simulink model "URM_IOKU_trajektorie_4_pokus"  (R2014a)
settings: Solver=ode45  StartTime=0.0  StopTime=3.975  MaxStep=1e-2  RelTol=1e-3
values from neighbouring files (symbols this model uses):
  a1 = 2    [URM_SP.m]
  a2 = 1.5    [URM_SP.m]
  a3 = 0.5    [URM_SP.m]
  D = linspace(d1,d2,n)    [URM_SP.m]
  vmax = 1    [URM_SP.m]
libraries: mblibv1 x12
settings Model: Creator=kajak_000  LastModifiedBy=kajak_000
settings SimMechanicsCC: VisDuringSimulation=on

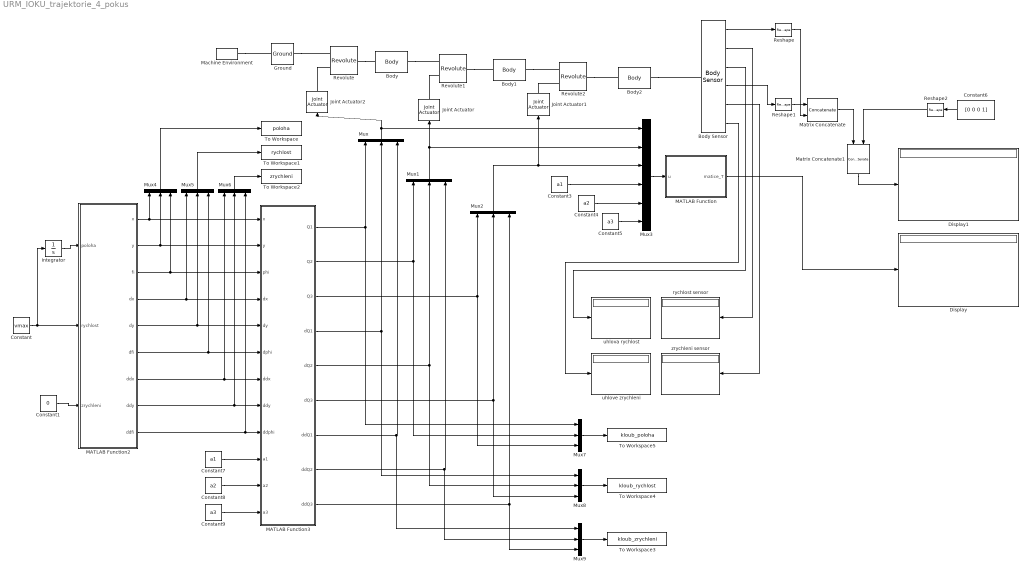
== system URM_IOKU_trajektorie_4_pokus ==
  Body : mblibv1/Bodies/Body  LConnTagsString=CS1  RConnTagsString=CS2  UpdateFromCAD=off  DialogClass=MechanicalBodyBlock  Mass=1  MassUnits=kg  InertiaUnits=kg*m^2  Inertia=eye(3)  Shape=Cylinder  ShapeDims=[1 1]  ShapeUnits=m  ShapeUse=false  Density=1  DensityUnits=kg/m^3  DensityUse=false  GraphicsMode=MACHINE_DEFAULT  BodyColorSelMode=MACHINE_DEFAULT  BodyColor=[1 0 0]  AttachedToCS=CG  CG=Left$CG$rameno1.CG$WORLD$WORLD$m$[0 0 0]$Euler X-Y-Z$deg$WORLD$false$none  WorkingFrames=Left$CS1$rameno1.A$World$World$m$[0 0 0]$Euler X-Y-Z$deg$WORLD$true$none#Right$CS2$rameno1.B$World$World$m$[0 0 0]$Euler X-Y-Z$deg$WORLD$true$none  CGPos=rameno1.CG  CGRot=[0 0 0]  CS0Pos=[]  CS0Rot=[]  CS1Pos=rameno1.A  CS1Rot=[0 0 0]  CS2Pos=rameno1.B  CS2Rot=[0 0 0]  CS3Pos=[]  CS3Rot=[]  CS4Pos=[]  CS4Rot=[]  CS5Pos=[]  CS5Rot=[]  CS6Pos=[]  CS6Rot=[]  CS7Pos=[]  CS7Rot=[]  CS8Pos=[]  CS8Rot=[]  CS9Pos=[]  CS9Rot=[]  CS10Pos=[]  CS10Rot=[]  CS11Pos=[]  CS11Rot=[]  CS12Pos=[]  CS12Rot=[]  CS13Pos=[]  CS13Rot=[]  CS14Pos=[]  CS14Rot=[]  CS15Pos=[]  CS15Rot=[]  CS16Pos=[]  CS16Rot=[]  CS17Pos=[]  CS17Rot=[]  CS18Pos=[]  CS18Rot=[]  CS19Pos=[]  CS19Rot=[]  CS20Pos=[]  CS20Rot=[]
  Body Sensor : mblibv1/Sensors &  Actuators/Body Sensor  UpdateFromCAD=off  PhysicalDomain=Mechanical  PortType=blob  Muxed=off  Pose=on  Angle=on  AngleUnits=deg  ArcVelocity=on  ArcVelocityUnits=rad/s  ArcAcceleration=on  ArcAccelerationUnits=rad/s^2  CoordPosition=on  CoordPositionUnits=m  Velocity=on  VelocityUnits=m/s  Acceleration=on  AccelerationUnits=m/s^2  Quaternion=on  QuaternionDT=off  QuaternionDDT=off  QuaternionUnits=off  OutputVector="[ 3  3  3  9  3  3]"  ActiveIO=on  Width=24  DialogClass=MechanicalSensorBlock  ReferenceFrame=Absolute (World)
  Body1 : mblibv1/Bodies/Body  LConnTagsString=CS1  RConnTagsString=CS2  UpdateFromCAD=off  DialogClass=MechanicalBodyBlock  Mass=1  MassUnits=kg  InertiaUnits=kg*m^2  Inertia=eye(3)  Shape=Cylinder  ShapeDims=[1 1]  ShapeUnits=m  ShapeUse=false  Density=1  DensityUnits=kg/m^3  DensityUse=false  GraphicsMode=MACHINE_DEFAULT  BodyColorSelMode=MACHINE_DEFAULT  BodyColor=[1 0 0]  AttachedToCS=CG  CG=Left$CG$rameno2.CG$WORLD$WORLD$m$[0 0 0]$Euler X-Y-Z$deg$WORLD$false$none  WorkingFrames=Left$CS1$rameno2.A$World$World$m$[0 0 0]$Euler X-Y-Z$deg$WORLD$true$none#Right$CS2$rameno2.B$World$World$m$[0 0 0]$Euler X-Y-Z$deg$WORLD$true$none  CGPos=rameno2.CG  CGRot=[0 0 0]  CS0Pos=[]  CS0Rot=[]  CS1Pos=rameno2.A  CS1Rot=[0 0 0]  CS2Pos=rameno2.B  CS2Rot=[0 0 0]  CS3Pos=[]  CS3Rot=[]  CS4Pos=[]  CS4Rot=[]  CS5Pos=[]  CS5Rot=[]  CS6Pos=[]  CS6Rot=[]  CS7Pos=[]  CS7Rot=[]  CS8Pos=[]  CS8Rot=[]  CS9Pos=[]  CS9Rot=[]  CS10Pos=[]  CS10Rot=[]  CS11Pos=[]  CS11Rot=[]  CS12Pos=[]  CS12Rot=[]  CS13Pos=[]  CS13Rot=[]  CS14Pos=[]  CS14Rot=[]  CS15Pos=[]  CS15Rot=[]  CS16Pos=[]  CS16Rot=[]  CS17Pos=[]  CS17Rot=[]  CS18Pos=[]  CS18Rot=[]  CS19Pos=[]  CS19Rot=[]  CS20Pos=[]  CS20Rot=[]
  Body2 : mblibv1/Bodies/Body  LConnTagsString=CS1  RConnTagsString=CS2  UpdateFromCAD=off  DialogClass=MechanicalBodyBlock  Mass=1  MassUnits=kg  InertiaUnits=kg*m^2  Inertia=eye(3)  Shape=Cylinder  ShapeDims=[1 1]  ShapeUnits=m  ShapeUse=false  Density=1  DensityUnits=kg/m^3  DensityUse=false  GraphicsMode=MACHINE_DEFAULT  BodyColorSelMode=MACHINE_DEFAULT  BodyColor=[1 0 0]  AttachedToCS=CG  CG=Left$CG$rameno3.CG$WORLD$WORLD$m$[0 0 0]$Euler X-Y-Z$deg$WORLD$false$none  WorkingFrames=Left$CS1$rameno3.A$World$World$m$[0 0 0]$Euler X-Y-Z$deg$WORLD$true$none#Right$CS2$rameno3.B$World$World$m$[0 0 0]$Euler X-Y-Z$deg$WORLD$true$none  CGPos=rameno3.CG  CGRot=[0 0 0]  CS0Pos=[]  CS0Rot=[]  CS1Pos=rameno3.A  CS1Rot=[0 0 0]  CS2Pos=rameno3.B  CS2Rot=[0 0 0]  CS3Pos=[]  CS3Rot=[]  CS4Pos=[]  CS4Rot=[]  CS5Pos=[]  CS5Rot=[]  CS6Pos=[]  CS6Rot=[]  CS7Pos=[]  CS7Rot=[]  CS8Pos=[]  CS8Rot=[]  CS9Pos=[]  CS9Rot=[]  CS10Pos=[]  CS10Rot=[]  CS11Pos=[]  CS11Rot=[]  CS12Pos=[]  CS12Rot=[]  CS13Pos=[]  CS13Rot=[]  CS14Pos=[]  CS14Rot=[]  CS15Pos=[]  CS15Rot=[]  CS16Pos=[]  CS16Rot=[]  CS17Pos=[]  CS17Rot=[]  CS18Pos=[]  CS18Rot=[]  CS19Pos=[]  CS19Rot=[]  CS20Pos=[]  CS20Rot=[]
  Constant : Constant  Value=vmax
  Constant1 : Constant  Value=0
  Constant3 : Constant  Value=a1
  Constant4 : Constant  Value=a2
  Constant5 : Constant  Value=a3
  Constant6 : Constant  Value=[0 0 0 1]
  Constant7 : Constant  Value=a1
  Constant8 : Constant  Value=a2
  Constant9 : Constant  Value=a3
  Display : Display
  Display1 : Display
  Ground : mblibv1/Bodies/Ground  UpdateFromCAD=off  LeftPortType=env  RightPortType=workingframe  PhysicalDomain=Mechanical  DialogClass=GroundBlock  CoordPosition=rameno1.A  CoordPositionUnits=m  StateVectorMgrId=0  MachineId=[1 0]  ShowEnvPort=on  ParameterChecksum=[1572609533, 1849027617, 4062556937, 1555680548]  TopologyChecksum=[3366249345, 1230097469, 3339338168, 2431679002]
  Integrator : Integrator
  Joint Actuator : mblibv1/Sensors &  Actuators/Joint Actuator  UpdateFromCAD=off  PhysicalDomain=Mechanical  PortType=blob  ActuationStyle=Motion  AngleUnits=rad  ArcVelocityUnits=rad/s  ArcAccelerationUnits=rad/s^2  CoordPositionUnits=m  VelocityUnits=m/s  AccelerationUnits=m/s^2  ForceUnits=N  TorqueUnits=N*m  ActiveIO=on  Width=3  DialogClass=MechanicalActuatorBlock  Primitive=R1  ReferenceFrame=Absolute (World)
  Joint Actuator1 : mblibv1/Sensors &  Actuators/Joint Actuator  UpdateFromCAD=off  PhysicalDomain=Mechanical  PortType=blob  ActuationStyle=Motion  AngleUnits=rad  ArcVelocityUnits=rad/s  ArcAccelerationUnits=rad/s^2  CoordPositionUnits=m  VelocityUnits=m/s  AccelerationUnits=m/s^2  ForceUnits=N  TorqueUnits=N*m  ActiveIO=on  Width=3  DialogClass=MechanicalActuatorBlock  Primitive=R1  ReferenceFrame=Absolute (World)
  Joint Actuator2 : mblibv1/Sensors &  Actuators/Joint Actuator  UpdateFromCAD=off  PhysicalDomain=Mechanical  PortType=blob  ActuationStyle=Motion  AngleUnits=rad  ArcVelocityUnits=rad/s  ArcAccelerationUnits=rad/s^2  CoordPositionUnits=m  VelocityUnits=m/s  AccelerationUnits=m/s^2  ForceUnits=N  TorqueUnits=N*m  ActiveIO=on  Width=3  DialogClass=MechanicalActuatorBlock  Primitive=R1  ReferenceFrame=Absolute (World)
  MATLAB Function : MATLAB Function  TreatAsAtomicUnit=on
  MATLAB Function2 : MATLAB Function  TreatAsAtomicUnit=on
  MATLAB Function3 : MATLAB Function  TreatAsAtomicUnit=on
  Machine Environment : mblibv1/Bodies/Machine Environment  PortType=env  PhysicalDomain=Mechanical  DialogTemplateClass=MECH.MachineEnvironment  SyncWhenCopied=off  Gravity=[0 0 0]  GravityUnits=m/s^2  GravityAsSignal=off  Dimensionality=Auto-detect  AnalysisType=Forward dynamics  LinearAssemblyTolerance=1e-3  LinearAssemblyToleranceUnits=m  AngularAssemblyTolerance=1e-3  AngularAssemblyToleranceUnits=rad  ConstraintSolverType=Stabilizing  ConstraintRelTolerance=1e-4  ConstraintAbsTolerance=1e-4  UseRobustSingularityHandling=off  RedundancyAnalysisToleranceType=Automatically select tolerance  RedundancyAnalysisTolerance=1e-14  StatePerturbationType=Fixed  PerturbationSize=1e-5  VisualizeMachine=on  BodyVisualizationType=Use model default body geometries  BodyColorSelMode=Use model default  DefaultBodyColor=[1 0 0]
  Matrix Concatenate : Concatenate  Mode=Multidimensional array  ConcatenateDimension=2
  Matrix Concatenate1 : Concatenate  Mode=Multidimensional array
  Mux{,1..2,4..9} (9 alike) : Mux  Inputs=3
  Mux3 : Mux  Inputs=6
  Reshape : Reshape  OutputDimensionality=Column vector (2-D)
  Reshape1 : Reshape  OutputDimensionality=Customize  OutputDimensions=[3,3]
  Reshape2 : Reshape  OutputDimensionality=Row vector (2-D)  OutputDimensions=[3,1]
  Revolute : mblibv1/Joints/Revolute  LConnTagsString=__newl0|SA1  RConnTagsString=__newr0  UpdateFromCAD=off  NumSAPorts=1  CutJoint=off  MarkAsCut=off  Primitives=prismatic  PrimitiveProps=R1$World$rameno1.osa$revolute  DialogClass=JointBlock  R1Axis=rameno1.osa
  Revolute1 : mblibv1/Joints/Revolute  LConnTagsString=__newl0|SA1  RConnTagsString=__newr0  UpdateFromCAD=off  NumSAPorts=1  CutJoint=off  MarkAsCut=off  Primitives=prismatic  PrimitiveProps=R1$World$rameno2.osa$revolute  DialogClass=JointBlock  R1Axis=rameno2.osa
  Revolute2 : mblibv1/Joints/Revolute  LConnTagsString=__newl0|SA1  RConnTagsString=__newr0  UpdateFromCAD=off  NumSAPorts=1  CutJoint=off  MarkAsCut=off  Primitives=prismatic  PrimitiveProps=R1$World$rameno3.osa$revolute  DialogClass=JointBlock  R1Axis=rameno3.osa
  To Workspace : ToWorkspace  VariableName=poloha  SaveFormat=Structure With Time  SampleTime=-1
  To Workspace1 : ToWorkspace  VariableName=rychlost  SaveFormat=Structure With Time  SampleTime=-1
  To Workspace2 : ToWorkspace  VariableName=zrychleni  SaveFormat=Structure With Time  SampleTime=-1
  To Workspace3 : ToWorkspace  VariableName=kloub_zrychleni  SaveFormat=Structure With Time  SampleTime=-1
  To Workspace4 : ToWorkspace  VariableName=kloub_rychlost  SaveFormat=Structure With Time  SampleTime=-1
  To Workspace5 : ToWorkspace  VariableName=kloub_poloha  SaveFormat=Structure With Time  SampleTime=-1
  rychlost sensor : Display
  uhlova rychlost : Display
  uhlove zrychleni : Display
  zrychleni sensor : Display
  wires:
  Constant3/1 -> Mux3/4
  Constant4/1 -> Mux3/5
  Constant5/1 -> Mux3/6
  Mux3/1 -> MATLAB Function/1(u)
  MATLAB Function/1(matice_T) -> Display/1
  Body Sensor/1 -> Reshape/1
  Body Sensor/4 -> Reshape1/1
  Reshape1/1 -> Matrix Concatenate/1
  Reshape/1 -> Matrix Concatenate/2
  Constant6/1 -> Reshape2/1
  Matrix Concatenate/1 -> Matrix Concatenate1/1
  Reshape2/1 -> Matrix Concatenate1/2
  Matrix Concatenate1/1 -> Display1/1
  Body Sensor/2 -> rychlost sensor/1
  Body Sensor/5 -> zrychleni sensor/1
  Body Sensor/3 -> uhlova rychlost/1
  Body Sensor/6 -> uhlove zrychleni/1
  Mux/1 -> Joint Actuator2/1, Mux3/1
  Mux1/1 -> Joint Actuator/1, Mux3/2
  Mux2/1 -> Joint Actuator1/1, Mux3/3
  Constant7/1 -> MATLAB Function3/10(a1)
  Constant8/1 -> MATLAB Function3/11(a2)
  Constant9/1 -> MATLAB Function3/12(a3)
  MATLAB Function3/1(Q1) -> Mux/1, Mux7/1
  MATLAB Function3/4(dQ1) -> Mux/2, Mux8/1
  MATLAB Function3/7(ddQ1) -> Mux9/1, Mux/3
  MATLAB Function3/2(Q2) -> Mux1/1, Mux7/2
  MATLAB Function3/5(dQ2) -> Mux1/2, Mux8/2
  MATLAB Function3/8(ddQ2) -> Mux9/2, Mux1/3
  MATLAB Function3/3(Q3) -> Mux2/1, Mux7/3
  MATLAB Function3/6(dQ3) -> Mux8/3, Mux2/2
  MATLAB Function3/9(ddQ3) -> Mux2/3, Mux9/3
  MATLAB Function2/1(x) -> MATLAB Function3/1(x), Mux4/1
  MATLAB Function2/2(y) -> MATLAB Function3/2(y), Mux4/2
  MATLAB Function2/3(fi) -> MATLAB Function3/3(phi), Mux4/3
  MATLAB Function2/4(dx) -> MATLAB Function3/4(dx), Mux5/1
  MATLAB Function2/5(dy) -> MATLAB Function3/5(dy), Mux5/2
  MATLAB Function2/6(dfi) -> MATLAB Function3/6(dphi), Mux5/3
  MATLAB Function2/7(ddx) -> MATLAB Function3/7(ddx), Mux6/1
  MATLAB Function2/8(ddy) -> MATLAB Function3/8(ddy), Mux6/2
  MATLAB Function2/9(ddfi) -> MATLAB Function3/9(ddphi), Mux6/3
  Integrator/1 -> MATLAB Function2/1(poloha)
  Constant/1 -> Integrator/1, MATLAB Function2/2(rychlost)
  Constant1/1 -> MATLAB Function2/3(zrychleni)
  Mux4/1 -> To Workspace/1
  Mux5/1 -> To Workspace1/1
  Mux6/1 -> To Workspace2/1
  Mux9/1 -> To Workspace3/1
  Mux8/1 -> To Workspace4/1
  Mux7/1 -> To Workspace5/1
  connections:
  Machine Environment/RConn1 -- Ground/LConn1
  Ground/RConn1 -- Revolute/LConn1
  Revolute/RConn1 -- Body/LConn1
  Body/RConn1 -- Revolute1/LConn1
  Revolute1/RConn1 -- Body1/LConn1
  Body1/RConn1 -- Revolute2/LConn1
  Revolute2/RConn1 -- Body2/LConn1
  Body2/RConn1 -- Body Sensor/LConn1
  Joint Actuator/RConn1 -- Revolute1/LConn2
  Joint Actuator1/RConn1 -- Revolute2/LConn2
  Joint Actuator2/RConn1 -- Revolute/LConn2

== matlab function URM_IOKU_trajektorie_4_pokus/MATLAB Function ==
  data: u input; matice_T output
function matice_T = DGM_funkce(u)
Q1 = u(1); % poloha
Q2 = u(4);
Q3 = u(7);
a1 = u(10);
a2 = u(11);
a3 = u(12);
matice_T = zeros(4);

x = a3 * cos(Q1 + Q2 + Q3) + a2 * cos(Q1 + Q2) + a1 * cos(Q1);
y = a3 * sin(Q1 + Q2 + Q3) + a2 * sin(Q1 + Q2) + a1 * sin(Q1);
vysledny_uhel = Q1 + Q2 + Q3; 

matice_T = [ cos(vysledny_uhel),-sin(vysledny_uhel),0,x;
            sin(vysledny_uhel),cos(vysledny_uhel),0,y;
            0,0,1,0;
            0,0,0,1 ];
       
end

== matlab function URM_IOKU_trajektorie_4_pokus/MATLAB Function2 ==
  data: x output; poloha input; y output; rychlost input; zrychleni input; fi output; dx output; dy output; dfi output; ddx output; ddy output; ddfi output
function [ x, y, fi, dx, dy, dfi, ddx, ddy, ddfi ] = trajektorie_funkce( poloha, rychlost, zrychleni )
% popis co je co
% x, y, fi pozadovana poloha + natoceni koncoveho efektoru
% dx, dy, dfi pozadovana rychlost + uhlova rychlost
% ddx, ddy, ddfi pozadovane zrychleni + uhlove zrychleni

% IOKU trajektorie
A = [2; 0.5]; 
B = [0; 1]; 
C = [2; 2.5]; 
r = 0.3; % polomer kruznice
vmax = 1;
dir = -1;

n_BA = (A - B)/ norm(A-B); % smerovy vektor z B do A
n_BC = (C - B)/ norm(C-B); % smerovy vektor z B do C
n_BS = (n_BA  + n_BC)/norm(n_BA  + n_BC); % smerovy vektor z B do S
K_1 = n_BA * n_BA' * n_BS - n_BS; 
l = r/(sqrt(K_1' * K_1)); % konstantni vzdalenost z B do S
S = B + n_BS * l; % souradnice stredu kruznice
k = n_BA' * (A - S); 

P_A = A - n_BA * k; % pocatecni bod oblouku
P_C = B + norm(P_A - B) * n_BC; %koncovy bod oblouku

dfi = acos((P_C - S)' * (P_A - S) / r^2); %delta phi
S_PA = (P_A - S);
fi_PA = atan2(S_PA(2), S_PA(1));

s1 = norm(P_A - A); % prvni usek - usecka
sk = r * dfi; %druhy usek - oblouk
s2 = norm(P_C - C); % treti usek - usecka

smax = s1 + sk + s2; % maximalni draha
tmax = smax/vmax; % maximalni cas

if poloha >=0 && poloha < s1
    k1 = poloha;
    dk1 = rychlost;
    ddk1 = zrychleni;
    X = [A - k1*n_BA; 0];
    dX = [-dk1 * n_BA; 0];
    ddX = [-ddk1 * n_BA; 0];
    
elseif s1 <= poloha && poloha < s1 + sk
    fi = (poloha - s1)/r;
    dfi = rychlost/r;
    ddfi = zrychleni/r;
    X = [r * [cos(fi_PA + dir * fi); sin(fi_PA + dir * fi)] + S; 0];
    dX = [r * [-sin(fi_PA + dir * fi); cos(fi_PA + dir * fi)] * dir * dfi; 0];
    ddX = [r * [-cos(fi_PA + dir * fi); -sin(fi_PA + dir * fi)] * dir^2 * dfi^2 + r * [-sin(fi_PA + dir * fi); cos(fi_PA + dir * fi)] * dir * ddfi; 0];
        
elseif s1 + sk <= poloha && poloha <= s1 + sk + s2
    k2 = poloha - s1 - sk;
    dk2 = rychlost;
    ddk2 = zrychleni;
    X = [P_C + k2*n_BC; 0];
    dX = [dk2 * n_BC; 0];
    ddX = [ddk2 * n_BC; 0];
else
   
    X = [0; 0; 0];
    dX = [0; 0; 0];
    ddX = [0; 0; 0];
end

x = X(1);
y = X(2);
fi = X(3);
dx = dX(1);
dy = dX(2);
dfi = dX(3);
ddx = ddX(1);
ddy = ddX(2);
ddfi = ddX(3);
end

== matlab function URM_IOKU_trajektorie_4_pokus/MATLAB Function3 ==
  data: Q1 output; Q2 output; Q3 output; dQ1 output; dQ2 output; dQ3 output; ddQ1 output; x input; y input; phi input; dx input; dy input; dphi input; ddx input; ddy input; ddphi input; a1 input; a2 input; a3 input; ddQ2 output; ddQ3 output
function [Q1, Q2, Q3, dQ1, dQ2, dQ3, ddQ1, ddQ2, ddQ3] = IOKU(x, y, phi, dx, dy, dphi, ddx, ddy, ddphi, a1, a2, a3)
%% vypocet Q2
cosQ2 = ((x - a3*cos(phi))^2 + (y - a3*sin(phi))^2 - a1^2 - a2^2)/(2 * a1 * a2);
sinQ2 = -abs(sqrt((1 - cosQ2^2))); %jeste zkontrolovat meze u slider gainu
Q2 = atan2(sinQ2, cosQ2);
%% vypocet Q1
A = [-a2 * sinQ2, a2 * cosQ2 + a1; a2 * cosQ2 + a1, a2 * sinQ2];
B = [x - a3*cos(phi); y - a3*sin(phi)];
v = A\B;
sinQ1 = v(1);
cosQ1 = v(2);
Q1 = atan2(sinQ1, cosQ1);
%% vypocet Q3
Q3 = phi - Q1 - Q2;
% rychlost dX
jQ = [-a3 * sin(Q1 + Q2 + Q3) - a2 * sin(Q1 + Q2) - a1 * sin(Q1), -a3 * sin(Q1 + Q2 + Q3) - a2 * sin(Q1 + Q2), -a3 * sin(Q1 + Q2 + Q3);...
    a3 * cos(Q1 + Q2 + Q3) + a2 * cos(Q1 + Q2) + a1 * cos(Q1), a3 * cos(Q1 + Q2 + Q3) + a2 * cos(Q1 + Q2), a3 * cos(Q1 + Q2 + Q3);...
    1, 1, 1];
dX = [dx; dy; dphi];
dQ = jQ^-1 * dX;
dQ1 = dQ(1);
dQ2 = dQ(2);
dQ3 = dQ(3);

% zrychleni ddX
djQ = [-a3*cos(Q1+Q2+Q3)*(dQ1+dQ2+dQ3) - a2*cos(Q1+Q2)*(dQ1+dQ2) - a1*cos(Q1)*dQ1, -a3*cos(Q1+Q2+Q3)*(dQ1+dQ2+dQ3) - a2*cos(Q1+Q2)*(dQ1+dQ2), -a3*cos(Q1+Q2+Q3)*(dQ1+dQ2+dQ3);...
    -a3*sin(Q1+Q2+Q3)*(dQ1+dQ2+dQ3) - a2*sin(Q1+Q2)*(dQ1+dQ2) - a1*sin(Q1)*dQ1, -a3*sin(Q1+Q2+Q3)*(dQ1+dQ2+dQ3) - a2*sin(Q1+Q2)*(dQ1+dQ2), -a3*sin(Q1+Q2+Q3)*(dQ1+dQ2+dQ3);...
    0, 0, 0];
ddX = [ddx; ddy; ddphi];
ddQ = jQ^-1 * (ddX - djQ * dQ);
ddQ1 = ddQ(1);
ddQ2 = ddQ(2);
ddQ3 = ddQ(3);
